simulink model "Vortex_flowmeter_simulation"  (R2020b)
settings: Solver=VariableStepAuto  StartTime=0.0  StopTime=0.05  MaxStep=0.00001  MinStep=0.000001  RelTol=1e-3
libraries: dspsigops x1
settings Model: Creator=GAURANG  LastModifiedBy=GAURANG
settings SolverCC: InitialStep=0.000001

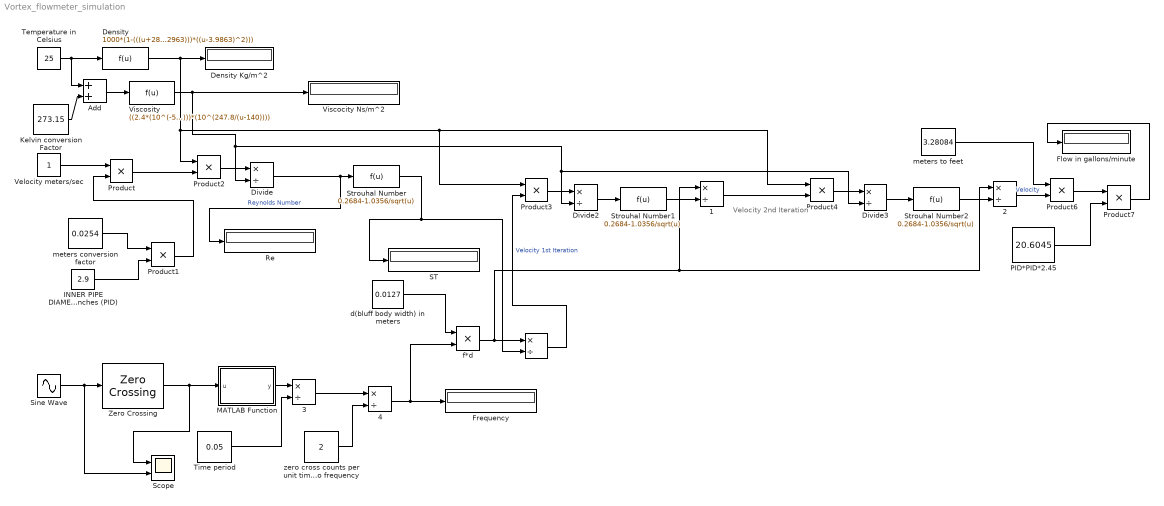
== system Vortex_flowmeter_simulation ==
  note: Velocity 2nd Iteration
   {,1..4} (5 alike) : Product  Inputs=*/
  Add : Sum
  "Density " : Fcn  Expr=1000*(1-(((u+288.9414)/((508929.2)*(u+68.12963)))*((u-3.9863)^2)))
  Density Kg/m^2 : Display
  Divide : Product  Inputs=*/
  Divide2 : Product  Inputs=*/
  Divide3 : Product  Inputs=*/
  "Flow in gallons/minute " : Display
  Frequency : Display
  INNER PIPE DIAMETER in inches (PID) : Constant  Value=2.9
  Kelvin conversion Factor : Constant  Value=273.15
  MATLAB Function : MATLAB Function  TreatAsAtomicUnit=on
  PID*PID*2.45 : Constant  Value=20.6045
  Product{,1..4,6..7} (7 alike) : Product
  Re : Display
  ST : Display
  Scope : Scope  NumInputPorts=2
  Sine Wave : Sin  Frequency=2*pi*250  SampleTime=0
  Strouhal Number : Fcn  Expr=0.2684-1.0356/sqrt(u)
  Strouhal Number1 : Fcn  Expr=0.2684-1.0356/sqrt(u)
  Strouhal Number2 : Fcn  Expr=0.2684-1.0356/sqrt(u)
  Temperature in Celsius : Constant  Value=25
  Time period : Constant  Value=0.05
  Velocity meters/sec : Constant
  Viscocity Ns/m^2 : Display
  Viscosity : Fcn  Expr=((2.4*(10^(-5)))*(10^(247.8/(u-140))))
  Zero Crossing : dspsigops/Zero Crossing
      settings: SourceProductBaseCode=DS
  d(bluff body width) in meters : Constant  Value=0.0127
  f*d : Product
  meters conversion factor : Constant  Value=0.0254
  "meters to feet " : Constant  Value=3.28084
  zero cross counts per unit time to frequency : Constant  Value=2
  wires:
  Temperature in Celsius/1 -> "Density "/1, Add/1
  Kelvin conversion Factor/1 -> Add/2
  Add/1 -> Viscosity/1
  "Density "/1 -> Product4/1, Product3/1, Product2/1, Density Kg/m^2/1
  Viscosity/1 -> Divide3/2, Divide2/2, Divide/2, Viscocity Ns/m^2/1
  INNER PIPE DIAMETER in inches (PID)/1 -> Product1/2
  meters conversion factor/1 -> Product1/1
  Product1/1 -> Product/2
  Product/1 -> Product2/2
  Product2/1 -> Divide/1
  Divide/1 -> Strouhal Number/1, Re/1  "Reynolds Number"
  Strouhal Number/1 -> " "/2, ST/1
  d(bluff body width) in meters/1 -> f*d/1
  f*d/1 -> " 2"/1, " 1"/1, " "/1
  " "/1 -> Product3/2  "Velocity 1st Iteration"
  Velocity meters/sec/1 -> Product/1
  Product3/1 -> Divide2/1
  Divide2/1 -> Strouhal Number1/1
  Strouhal Number1/1 -> " 1"/2
  " 1"/1 -> Product4/2
  Product4/1 -> Divide3/1
  Divide3/1 -> Strouhal Number2/1
  Strouhal Number2/1 -> " 2"/2
  "meters to feet "/1 -> Product6/1
  Product6/1 -> Product7/1
  PID*PID*2.45/1 -> Product7/2
  Product7/1 -> "Flow in gallons/minute "/1
  " 2"/1 -> Product6/2  "Velocity"
  Sine Wave/1 -> Zero Crossing/1, Scope/2
  Zero Crossing/1 -> MATLAB Function/1(u), Scope/1
  Time period/1 -> " 3"/2
  MATLAB Function/1(y) -> " 3"/1
  " 3"/1 -> " 4"/1
  zero cross counts per unit time to frequency/1 -> " 4"/2
  " 4"/1 -> Frequency/1, f*d/2

== matlab function Vortex_flowmeter_simulation/MATLAB Function ==
  data: u input; y output
function y = fcn(u)
persistent count1
if isempty(count1)
    count1= 0
end
if u > 0
    count1=count1+1
end
y = count1;
